simulink model "CSTR_Open"  (R2021a)
settings: Solver=VariableStepAuto  StartTime=0.0  StopTime=20  RelTol=1e-3
values from neighbouring files (symbols this model uses):
  caf = 10    [mainCSTR.m]    (also in mainCSTR_control.m; mainControlCSTR.m; simulation_04_04_2024.mat)
  deltaE = 11843    [mainCSTR.m]    (also in mainCSTR_control.m; mainControlCSTR.m; simulation_04_04_2024.mat)
  deltaH = 5960    [mainCSTR.m]    (also in mainCSTR_control.m; mainControlCSTR.m; simulation_04_04_2024.mat)
  fov = fov0(i)    [mainCSTR_control.m]    (also in mainControlCSTR.m; reator_cstr.m = u(1))
  k0 = 9703*3600    (= 34930800)    [mainCSTR.m]    (also in mainCSTR_control.m; mainControlCSTR.m; simulation_04_04_2024.mat)
  R = 1.987    [mainCSTR.m]    (also in mainCSTR_control.m; mainControlCSTR.m; rga.m = pinv(G.').*G; simulation_04_04_2024.mat)
  rhocp = 500    [mainCSTR.m]    (also in mainCSTR_control.m; mainControlCSTR.m; simulation_04_04_2024.mat)
  Tc = Tc0(i)    [mainCSTR_control.m]    (also in mainControlCSTR.m; reator_cstr.m = u(2))
  Tf = 298    [mainCSTR.m]    (also in mainCSTR_control.m; mainControlCSTR.m; simulation_04_04_2024.mat)
  Ts = 0.1    [mainCSTR_control.m]    (also in mainControlCSTR.m; wandb.m = 0.5)
  UAoV = 150    [mainCSTR.m]    (also in mainCSTR_control.m; mainControlCSTR.m; simulation_04_04_2024.mat)
  x0model = [5, 350]    [mainCSTR.m]    (also in mainCSTR_control.m = [8.5636  311.1710]; mainControlCSTR.m = [8.5636  311.1706]; simulation_04_04_2024.mat = [5 350])
settings Model: Creator=Aula  LastModifiedBy=Aula
settings DataIOCC: ReturnWorkspaceOutputs=off

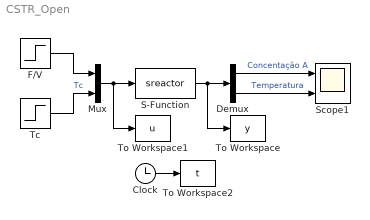
== system CSTR_Open ==
  Clock : Clock
  Demux : Demux  Outputs=2
  F/V : Step  Time=0  After=fov  SampleTime=0
  Mux : Mux  Inputs=2
  S-Function : S-Function  FunctionName=sreactor  Parameters=x0model,k0,deltaE,R,caf,Tf,deltaH,rhocp,UAoV  SFunctionDeploymentMode=off  EnableBusSupport=off
  Scope1 : Scope  NumInputPorts=2
  Tc : Step  Time=0  After=Tc  SampleTime=0
  To Workspace : ToWorkspace  VariableName=y  SampleTime=Ts
  "To Workspace1 " : ToWorkspace  VariableName=u  SampleTime=Ts
  "To Workspace2 " : ToWorkspace  VariableName=t  SampleTime=Ts
  wires:
  Clock/1 -> "To Workspace2 "/1
  Demux/2 -> Scope1/2  "Temperatura"
  Demux/1 -> Scope1/1  "Concentação A"
  S-Function/1 -> Demux/1, To Workspace/1
  Mux/1 -> S-Function/1, "To Workspace1 "/1
  F/V/1 -> Mux/1
  Tc/1 -> Mux/2  "Tc"
